simulink model "pendulem_sim"  (R2023a)
settings: Solver=ode1  StartTime=0.0  StopTime=10.0  FixedStep=0.001  MaxStep=0.001  RelTol=1e-3
values from neighbouring files (symbols this model uses):
  A = [ 0 1 0 0 ... (first row only)    [part4.m]    (also in untitled2.m = [1;0])
  B = [ 0; -0.87; 0; 163]    [part4.m]
  C = [1 0 0 0 ; 0 0 1 0]    [part4.m]
undefined symbols (not defined in the file or in its folder): L
libraries: fricblocks x1
settings Model: Creator=rawnies2  LastModifiedBy=rawnies2

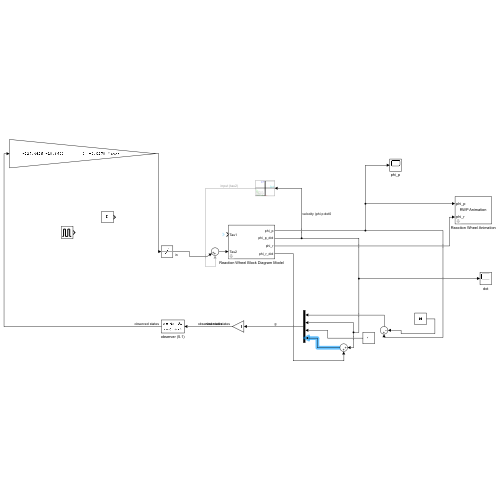
[thumbnail: Simulink's stored preview of the top-level diagram]
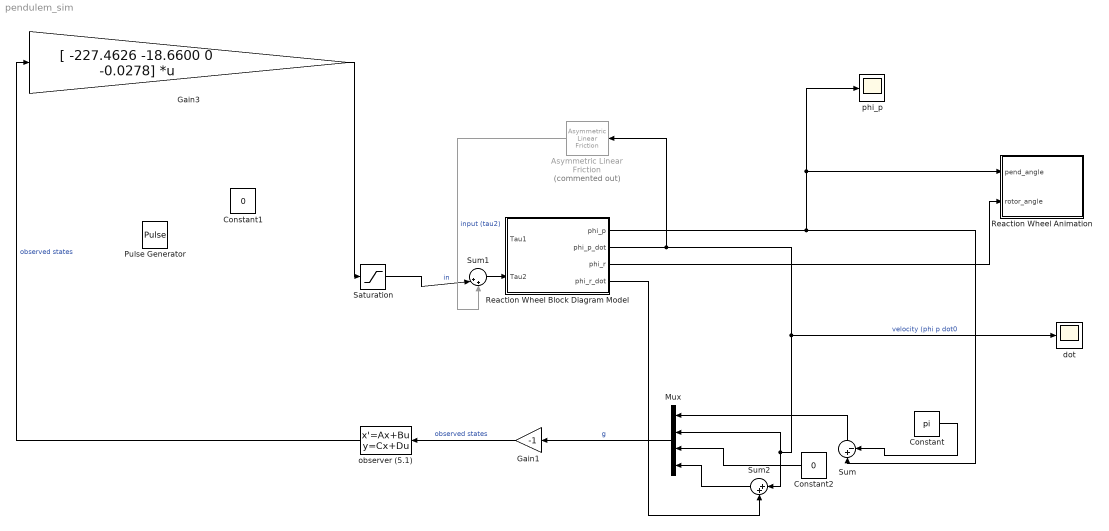
== system pendulem_sim ==
  Asymmetric Linear Friction : fricblocks/Asymmetric  Linear Friction  Commented=on  intercept1=0.6043  intercept2=-0.6143  slope1=0.01219  slope2=0.01291
  Constant : Constant  Value=pi
  Constant1 : Constant  Value=0
  Constant2 : Constant  Value=0
  Gain1 : Gain  Gain=-1
  Gain3 : Gain  Gain="[ -227.4626  -18.6600   0   -0.0278]"  Multiplication=Matrix(K*u) (u vector)
  Mux : Mux
  Pulse Generator : DiscretePulseGenerator  PulseType=Time based  Amplitude=8  Period=4  PulseWidth=5
  Reaction Wheel Animation : Subsystem  mask(Reaction Wheel Animation){}
      mask help: The animation block takes as input the pendulum angle (in radians), with 0 pointing down. Use this to visualize the pendulum position while testing controllers.
      mask Help: The animation block takes as input the pendulum angle (in radians), with 0 pointing down.  Use this to visualize the pendulum position while testing controllers.
      mask Display:
      | port_label('input', 1, 'phi_p')
      | port_label('input', 2, 'phi_r')
      | fprintf('RWP Animation')
  Reaction Wheel Block Diagram Model : Subsystem  mask(Reaction Wheel Block Diagram Model){par=[77.6 0.87 163], g=9.804, init=[pi+0.4 0 0 0]}
      mask prompts: par "Internal Parameters (a, bp, br)"; g "Acceleration of Gravity"; init "Initial Conditions"
      mask help:
      | This is a <i>nonlinear mathematical model</i> of the reaction wheel pendulum.  It takes as inputs torques to the system, and outputs a state vector.
      | <p>
      | <h2>Parameters</h2>
      | <ul>
      | <h3>Internal Parameters</h3>
      | <ul>
      | <li><b>a</b>, the square of the frquency of small oscillations ( a = omega<sub>p</sub><sup>2</sup>) </li>
      | <li><b>b<sub>p</sub></b>, the control gain over total inertia (b<sub>p</sub> = k<sub>u</sub>/J)</li>
      | <li><b>b<sub>r</sub></b>, the control gain over rotor inertia (b<sub>r</sub> = k<sub>u</sub>/J<sub>r</sub>)</li>
      | </ul>
      | <h3>Acceleration of Gravity</h3>
      | <ul>
      | <li><b>g</b>, commonly 9.804</li>
      | </ul>
      | <h3>Initial Conditions</h3>
      | Starting values for the state vector.  Usually, use [pi, 0,0,0] to start the pendulum at rest in the unstable equilibrium position pointing upwards.
      | <ul>
      | <li><b>phi<sub>p</sub></b>, encoder angle of the pendulum, in radians (0 is down)</li>
      | <li><b>phi<sub>p</sub>dot</b>, angular velocity of the pendulum, in radians/sec</li>
      | <li><b>phi<sub>r</sub></b>, encoder angle of the rotor, in radians (0 is down)</li>
      | <li><b>phi<sub>r</sub>dot</b>, angular velocity of the pendulum, in radians/sec</li>
      | </ul>
      | </ul>
      | <p>
      mask Help:
      | This is a <i>nonlinear mathematical model</i>  of the reaction wheel pendulum.  It takes as inputs torques to the system, and outputs a state vector.
      | <p>
      | <h2>Parameters</h2>
      | <ul>
      | <h3>Internal Parameters</h3>
      | <ul>
      | <li><b>a</b>, the square of the frquency of small oscillations ( a = omega<sub>p</sub><sup>2</sup>) </li>
      | <li><b>b<sub>p</sub></b>, the control gain over total inertia (b<sub>p</sub> = k<sub>u</sub>/J)</li>
      | <li><b>b<sub>r</sub></b>, the control gain over rotor inertia (b<sub>r</sub> = k<sub>u</sub>/J<sub>r</sub>)</li>
      | </ul>
      | <h3>Acceleration of Gravity</h3>
      | <ul>
      | <li><b>g</b>, commonly 9.804</li>
      | </ul>
      | <h3>Initial Conditions</h3>
      | Starting values for the state vector.  Usually, use [pi, 0,0,0] to start the pendulum at rest in the unstable equilibrium position pointing upwards.
      | <ul>
      | <li><b>phi<sub>p</sub></b>, encoder angle of the pendulum, in radians (0 is down)</li>
      | <li><b>phi<sub>p</sub>dot</b>, angular velocity of the pendulum, in radians/sec</li>
      | <li><b>phi<sub>r</sub></b>, encoder angle of the rotor, in radians (0 is down)</li>
      | <li><b>phi<sub>r</sub>dot</b>, angular velocity of the pendulum, in radians/sec</li>
      | </ul>
      | </ul>
      | <p>
      | 
      | <h2>Inputs</h2>
      | <ul>
      | <li><b>Tau1</b>, external force on the pendulum arm. (This arm is not actuated, but disturbances can be applied here)</li>
      | <li><b>Tau2</b>, external force on the rotor.  (input to the motor + disturbances)</li>
      | </ul>
      | 
      | <h2>Outputs</h2>
      | <ul>
      |  Outputs the current state vector. (See Initial Conditions)
      | </ul>
      | <p>
      | Don’t forget to include a Saturation block (to saturate the control effort at +/- 10) before <i>Tau2</i>.
      | <p>
      | <!-- last updates, Summer, 2007 -->
  Saturation : Saturate  UpperLimit=10  LowerLimit=-10
  Sum : Sum  Inputs=|+-
  Sum1 : Sum  Inputs=||++
  Sum2 : Sum  Inputs=|++
  dot : Scope
  observer (5.1) : StateSpace  A=A-L*C  B=[B L]  C=eye(4)  D=zeros(4, 3)  InitialCondition=0  ParameterTunability=Unconstrained
  phi_p : Scope
  wires:
  Reaction Wheel Block Diagram Model/1(phi_p) -> Sum/1, phi_p/1, Reaction Wheel Animation/1(pend_angle)
  Mux/1 -> Gain1/1  "g"
  Gain3/1 -> Saturation/1
  Reaction Wheel Block Diagram Model/2(phi_p_dot) -> Asymmetric Linear Friction/1, Sum2/1, Mux/2, dot/1  "velocity (phi p dot0"
  Sum/1 -> Mux/1
  Reaction Wheel Block Diagram Model/3(phi_r) -> Reaction Wheel Animation/2(rotor_angle)
  Constant/1 -> Sum/2
  Saturation/1 -> Sum1/1  "in"
  Sum1/1 -> Reaction Wheel Block Diagram Model/2(Tau2)
  Asymmetric Linear Friction/1 -> Sum1/2  "input (tau2)"
  Constant2/1 -> Mux/3
  Reaction Wheel Block Diagram Model/4(phi_r_dot) -> Sum2/2
  Sum2/1 -> Mux/4
  Gain1/1 -> observer (5.1)/1  "observed states"
  observer (5.1)/1 -> Gain3/1  "observed states"

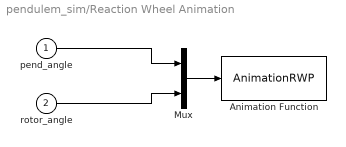
== system pendulem_sim/Reaction Wheel Animation ==
  pend_angle : Inport
  rotor_angle : Inport  Port=2
  Animation Function : S-Function  FunctionName=AnimationRWP  Parameters=0.05  SFunctionDeploymentMode=off  EnableBusSupport=off
      settings: DeleteFcn=if ~isempty(findobj('type','figure','name','dblpend1 Animation'));close('dblpend1 Animation'); end;
  Mux : Mux  Inputs=2
  wires:
  Mux/1 -> Animation Function/1
  rotor_angle/1 -> Mux/2
  pend_angle/1 -> Mux/1

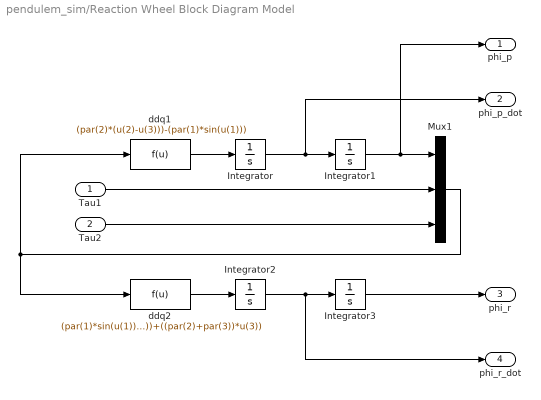
== system pendulem_sim/Reaction Wheel Block Diagram Model ==
  Tau1 : Inport
  Tau2 : Inport  Port=2
  Integrator : Integrator  InitialCondition=init(2)
  Integrator1 : Integrator  InitialCondition=init(1)
  Integrator2 : Integrator  InitialCondition=init(4)
  Integrator3 : Integrator  InitialCondition=init(3)
  Mux1 : Mux  Inputs=3
  ddq1 : Fcn  Expr=(par(2)*(u(2)-u(3)))-(par(1)*sin(u(1)))
  ddq2 : Fcn  Expr=(par(1)*sin(u(1)))-(par(2)*u(2))+((par(2)+par(3))*u(3))
  phi_p : Outport
  phi_p_dot : Outport  Port=2
  phi_r : Outport  Port=3
  phi_r_dot : Outport  Port=4
  wires:
  Mux1/1 -> ddq1/1, ddq2/1
  Tau2/1 -> Mux1/3
  Tau1/1 -> Mux1/2
  Integrator1/1 -> Mux1/1, phi_p/1
  Integrator/1 -> Integrator1/1, phi_p_dot/1
  Integrator2/1 -> Integrator3/1, phi_r_dot/1
  Integrator3/1 -> phi_r/1
  ddq2/1 -> Integrator2/1
  ddq1/1 -> Integrator/1
